simulink model "BAM"  (R2025b)
settings: Solver=FixedStepAuto  StartTime=0.0  StopTime=SimPar.model_params.stop_time  RelTol=1e-3
libraries: simulink x1, ros2lib x1
settings Model: Creator=macheson  LastModifiedBy=Ethan Dueck

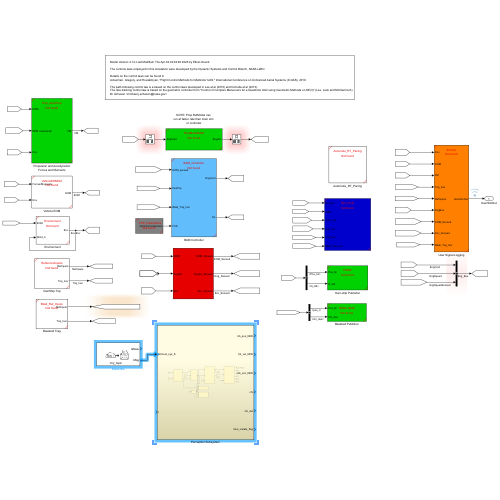
[thumbnail: Simulink's stored preview of the top-level diagram]
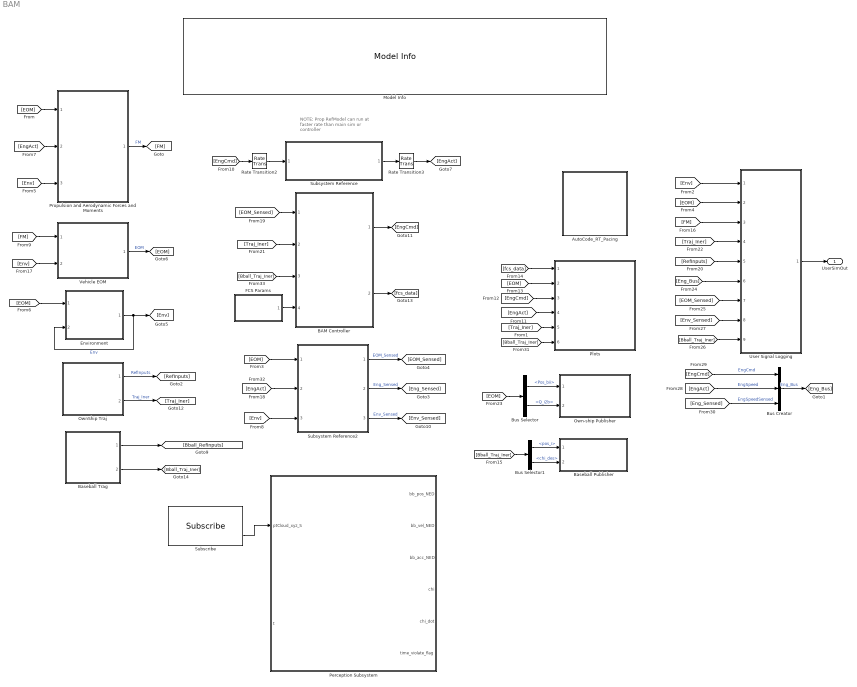
== system BAM ==
  note: NOTE: Prop RefModel can
      | run at faster rate than main sim
      | or controller
  AutoCode_RT_Pacing : Subsystem  ReferencedSubsystem=Autocode_RT_Pacing
  BAM Controller : Subsystem  ReferencedSubsystem=BAM_Controller
  Baseball Publisher : Subsystem  ReferencedSubsystem=ROS2_Bball
  Baseball Trag : Subsystem  ReferencedSubsystem=Bball_Ref_Inputs
  Bus Creator : BusCreator  Inputs=3  OutDataTypeStr=Bus: BUS_PROP_CMD
  Bus Selector : BusSelector  OutputSignals=InertialData.Pos_bii,InertialData.Q_i2b
  Bus Selector1 : BusSelector  OutputSignals=pos_i,chi_des
  Environment : Subsystem  ReferencedSubsystem=Environment
  FCS Params : Subsystem  ReferencedSubsystem=FCS_Parameters
  Model Info : simulink/Model-Wide Utilities/Model Info  Frame=on  DisplayStringWithTags=|  HorizontalTextAlignment=Left  LeftAlignmentValue=0.02
      | Model Version %<ModelVersion>; Last Modified: %<LastModificationDate> by %<LastModifiedBy>
      | 
      | The controls laws employed in this simulation were developed by the Dynamic Systems and Control Branch, NASA LaRC.
      | 
      | Details on the control laws can be found in
      | Ackerman, Gregory, and Hovakimyan, "Flight Control Methods for Multirotor UAS," International Conference on Unmanned Aerial Systems (ICUAS), 2019.
      | 
      | The path-following control law is a based on the control laws developed in Lee et al (2010) and Cichella et al (2013). 
      | The rate-tracking control law is based on the geometric controller from "Control of Complex Maneuvers for a Quadrotor UAV using Geometric Methods on SE(3)" (Lee, Leok and McClamroch)
      | M. Acheson <michael.j.acheson@nasa.gov>
  Own-ship Publisher : Subsystem  ReferencedSubsystem=ROS2
  OwnShip Traj : Subsystem  ReferencedSubsystem=ReferenceInputs
  Perception Subsystem : Subsystem
  Plots : Subsystem  ReferencedSubsystem=Sim_Plots
  Propulsion and Aerodynamic Forces and Moments : Subsystem  ReferencedSubsystem=Poly_AeroProp
  Rate Transition2 : RateTransition  OutPortSampleTime=SimIn.model_params.sim_rate
  Rate Transition3 : RateTransition  OutPortSampleTime=SimIn.model_params.sim_rate
  Subscribe : ros2lib/Subscribe  topicSource=Select from ROS network  topic=/my_topic  messageType=geometry_msgs/Point  sampleTime=-1  QOSHistory=Keep last  QOSDepth=10  QOSReliability=Reliable  QOSDurability=Volatile  QOSDeadline=Inf  QOSLifespan=Inf  QOSLiveliness=Automatic  QOSLeaseDuration=Inf  QOSAvoidROSNamespaceConventions=off
  Subsystem Reference : Subsystem  ReferencedSubsystem=PropModelBAM
  Subsystem Reference2 : Subsystem  ReferencedSubsystem=Sensors
  User Signal Logging : Subsystem  ReferencedSubsystem=SimOut
  Vehicle EOM : Subsystem  ReferencedSubsystem=VehicleEOMRef
  UserSimOut : Outport
  wires:
  Vehicle EOM/1 -> [EOM]  "EOM"
  [FM] -> Vehicle EOM/1
  [Env] -> Vehicle EOM/2
  [EOM] -> Propulsion and Aerodynamic Forces and Moments/1
  OwnShip Traj/1 -> [RefInputs]  "RefInputs"
  Propulsion and Aerodynamic Forces and Moments/1 -> [FM]  "FM"
  [EOM] -> Subsystem Reference2/1
  Environment/1 -> Environment/2, [Env]  "Env"
  [EOM] -> Environment/1
  Subsystem Reference/1 -> Rate Transition3/1
  [EngCmd] -> Rate Transition2/1
  [EngAct] -> Plots/4
  [EngCmd] -> Plots/3
  [EOM] -> Plots/2
  [fcs_data] -> Plots/1
  [EngAct] -> Propulsion and Aerodynamic Forces and Moments/2
  Rate Transition2/1 -> Subsystem Reference/1
  Rate Transition3/1 -> [EngAct]
  Subsystem Reference2/2 -> [Eng_Sensed]  "Eng_Sensed"
  Subsystem Reference2/3 -> [Env_Sensed]  "Env_Sensed"
  [Env] -> Subsystem Reference2/3
  [EngAct] -> Subsystem Reference2/2
  Subsystem Reference2/1 -> [EOM_Sensed]  "EOM_Sensed"
  FCS Params/1 -> BAM Controller/4
  [EOM_Sensed] -> BAM Controller/1
  [Traj_Iner] -> BAM Controller/2
  BAM Controller/1 -> [EngCmd]
  OwnShip Traj/2 -> [Traj_Iner]  "Traj_Iner"
  BAM Controller/2 -> [fcs_data]
  [Env] -> User Signal Logging/1
  [EOM] -> User Signal Logging/2
  [Env_Sensed] -> User Signal Logging/8
  [EOM_Sensed] -> User Signal Logging/7
  [Eng_Bus] -> User Signal Logging/6
  [Traj_Iner] -> User Signal Logging/4
  [RefInputs] -> User Signal Logging/5
  [FM] -> User Signal Logging/3
  Bus Creator/1 -> [Eng_Bus]  "Eng_Bus"
  [Eng_Sensed] -> Bus Creator/3  "EngSpeedSensed"
  [EngAct] -> Bus Creator/2  "EngSpeed"
  [EngCmd] -> Bus Creator/1  "EngCmd"
  [EOM] -> Bus Selector/1
  Bus Selector/1 -> Own-ship Publisher/1  "<Pos_bii>"
  Bus Selector/2 -> Own-ship Publisher/2  "<Q_i2b>"
  User Signal Logging/1 -> UserSimOut/1
  [Traj_Iner] -> Plots/5
  Baseball Trag/1 -> [Bball_RefInputs]
  Baseball Trag/2 -> [Bball_Traj_Iner]
  [Bball_Traj_Iner] -> Plots/6
  [Bball_Traj_Iner] -> User Signal Logging/9
  [Bball_Traj_Iner] -> Bus Selector1/1
  Bus Selector1/1 -> Baseball Publisher/1  "<pos_i>"
  Bus Selector1/2 -> Baseball Publisher/2  "<chi_des>"
  [Env] -> Propulsion and Aerodynamic Forces and Moments/3
  [Bball_Traj_Iner] -> BAM Controller/3
  Subscribe/2 -> Perception Subsystem/1(ptCloud_xyz_S)

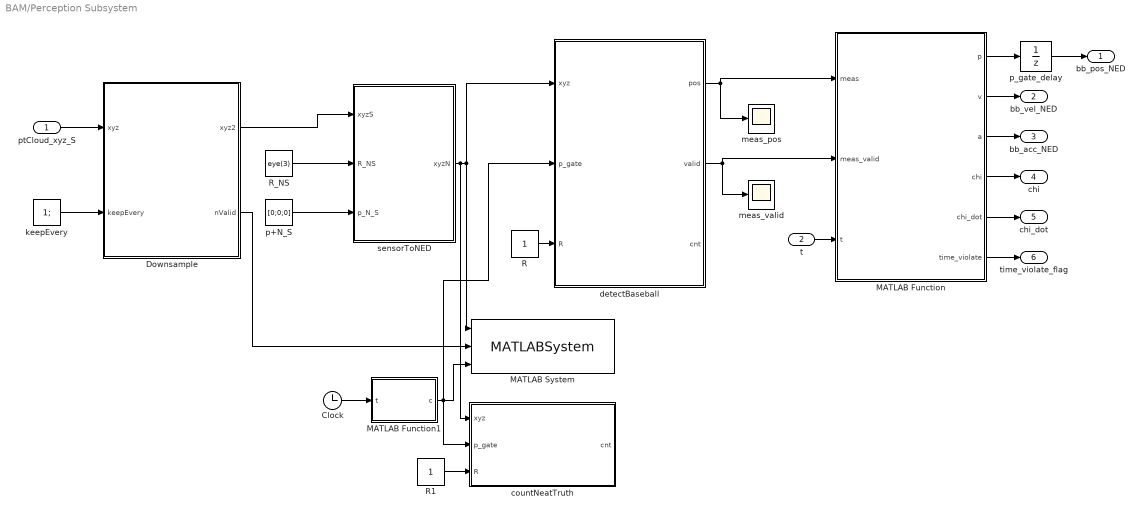
== system BAM/Perception Subsystem ==
  ptCloud_xyz_S : Inport
  t : Inport  Port=2
  Clock : Clock
  Downsample : MATLAB Function  TreatAsAtomicUnit=on
  MATLAB Function : MATLAB Function  TreatAsAtomicUnit=on
  MATLAB Function1 : MATLAB Function  TreatAsAtomicUnit=on
  MATLAB System : MATLABSystem  System=PointCloudViewer  PointSize=3  XLim=[0 60]  YLim=[-30 30]  ZLim=[-10 10]  Decimate=5  ShowDetection=on  SimulateUsing=Interpreted execution
      mask Type: PointCloudViewer
  R : Constant
  R1 : Constant
  R_NS : Constant  Value=eye(3)
  countNeatTruth : MATLAB Function  TreatAsAtomicUnit=on
  detectBaseball : MATLAB Function  TreatAsAtomicUnit=on
  keepEvery : Constant  Value=1;
  meas_pos : Scope
      settings: ActiveDisplayYMinimum=-16.997474195338938  ActiveDisplayYMaximum=39.269494336463588
  meas_valid : Scope
      settings: ActiveDisplayYMinimum=0.9  ActiveDisplayYMaximum=1.1  DataLoggingVariableName=ScopeData4
  p+N_S : Constant  Value=[0;0;0]
  p_gate_delay : UnitDelay  InitialCondition=[10; 0; -2]  SampleTime=-1  HasFrameUpgradeWarning=on
  sensorToNED : MATLAB Function  TreatAsAtomicUnit=on
  bb_pos_NED : Outport
  bb_vel_NED : Outport  Port=2
  bb_acc_NED : Outport  Port=3
  chi : Outport  Port=4
  chi_dot : Outport  Port=5
  time_violate_flag : Outport  Port=6
  wires:
  MATLAB Function/2(v) -> bb_vel_NED/1
  MATLAB Function/3(a) -> bb_acc_NED/1
  MATLAB Function/4(chi) -> chi/1
  MATLAB Function/5(chi_dot) -> chi_dot/1
  MATLAB Function/6(time_violate) -> time_violate_flag/1
  t/1 -> MATLAB Function/3(t)
  detectBaseball/2(valid) -> MATLAB Function/2(meas_valid), meas_valid/1
  R_NS/1 -> sensorToNED/2(R_NS)
  ptCloud_xyz_S/1 -> Downsample/1(xyz)
  Downsample/1(xyz2) -> sensorToNED/1(xyzS)
  keepEvery/1 -> Downsample/2(keepEvery)
  p+N_S/1 -> sensorToNED/3(p_N_S)
  MATLAB Function/1(p) -> p_gate_delay/1
  p_gate_delay/1 -> bb_pos_NED/1
  sensorToNED/1(xyzN) -> countNeatTruth/1(xyz), detectBaseball/1(xyz), MATLAB System/1
  Downsample/2(nValid) -> MATLAB System/2
  detectBaseball/1(pos) -> meas_pos/1, MATLAB Function/1(meas)
  Clock/1 -> MATLAB Function1/1(t)
  MATLAB Function1/1(c) -> detectBaseball/2(p_gate), countNeatTruth/2(p_gate), MATLAB System/3
  R/1 -> detectBaseball/3(R)
  R1/1 -> countNeatTruth/3(R)

== matlab function BAM/Perception Subsystem/sensorToNED ==
  data: xyzS input; xyzN output; R_NS input; p_N_S input
function xyzN = sensorToNED(xyzS, R_NS, p_N_S)
%#codegen
N = size(xyzS,1);
xyzN = zeros(N,3,'like',xyzS);

for i = 1:N
    p = xyzS(i,:).';
    if ~all(isfinite(p))
        xyzN(i,:) = [NaN NaN NaN];
    else
        q = R_NS*p + p_N_S;
        xyzN(i,:) = q.';
    end
end
end

== matlab function BAM/Perception Subsystem/Downsample ==
  data: xyz input; xyz2 output; keepEvery input; nValid output
function [xyz2, nValid] = Downsample(xyz, keepEvery)
%#codegen
N = int32(size(xyz,1));          % should be 11520
xyz2 = zeros(double(N),3,'like',xyz);

nValid = int32(0);

k = int32(keepEvery);
if k < 1
    k = int32(1);
end

% Fill with NaNs (viewer will drop them; avoids axis blow-up)
nanv = cast(NaN,'like',xyz);
xyz2(:,:) = nanv;

j = int32(0);
for i = int32(1):k:N
    j = j + 1;
    xyz2(double(j),:) = xyz(double(i),:);
end

nValid = j;
end

== matlab function BAM/Perception Subsystem/MATLAB Function1 ==
  data: t input; c output
function c = ballTruth(t)
%#codegen
c = [30; 0.5*t; -2];
end

== matlab function BAM/Perception Subsystem/countNeatTruth ==
  data: xyz input; cnt output; p_gate input; R input
function cnt = countNearTruth(xyz, p_gate, R)
%#codegen
cnt = int32(0);
R2 = double(R)*double(R);

N = size(xyz,1);
for i = 1:N
    n = xyz(i,1); e = xyz(i,2); d = xyz(i,3);
    if ~isfinite(n) || ~isfinite(e) || ~isfinite(d)
        continue;
    end
    dn = n - p_gate(1);
    de = e - p_gate(2);
    dd = d - p_gate(3);
    if (dn*dn + de*de + dd*dd) <= R2
        cnt = cnt + 1;
    end
end
end

== matlab function BAM/Perception Subsystem/detectBaseball ==
  data: xyz input; pos output; valid output; cnt output; p_gate input; R input
function [pos, valid, cnt] = detectBallSphereGate(xyz, p_gate, R)
%#codegen
pos   = zeros(3,1);
valid = false;
cnt   = int32(0);

R2 = double(R)*double(R);
s  = zeros(3,1);

N = size(xyz,1);
for i = 1:N
    n = xyz(i,1); e = xyz(i,2); d = xyz(i,3);
    if ~isfinite(n) || ~isfinite(e) || ~isfinite(d)
        continue;
    end

    dn = n - p_gate(1);
    de = e - p_gate(2);
    dd = d - p_gate(3);

    if (dn*dn + de*de + dd*dd) <= R2
        cnt = cnt + 1;
        s = s + [n; e; d];
    end
end

if cnt >= 5
    pos = s / double(cnt);
    valid = true;
end
end

== matlab function BAM/Perception Subsystem/MATLAB Function ==
  data: meas input; p output; meas_valid input; t input; v output; a output; chi output; chi_dot output; time_violate output
function [p,v,a,chi,chi_dot,time_violate] = trackBaseball(meas, meas_valid, t)
%#codegen

persistent p_hat v_hat a_hat t_last t_meas_last init

if isempty(init)
    p_hat = zeros(3,1);
    v_hat = zeros(3,1);
    a_hat = zeros(3,1);
    t_last = t;
    t_meas_last = t;     % <-- avoid -Inf
    init = true;
end

% Guard against time going backwards or being constant
dt_raw = t - t_last;
if ~isfinite(dt_raw) || dt_raw <= 0
    dt = 1e-3;
else
    dt = dt_raw;
end
t_last = t;

% prediction
p_hat = p_hat + v_hat*dt + 0.5*a_hat*(dt*dt);
v_hat = v_hat + a_hat*dt;

% update (alpha-beta-gamma)
alpha = 0.7; beta = 0.2; gamma = 0.05;

meas_ok = meas_valid && all(isfinite(meas(:)));

if meas_ok
    r = meas - p_hat;
    p_hat = p_hat + alpha*r;
    v_hat = v_hat + (beta/dt)*r;
    a_hat = a_hat + (2*gamma/(dt*dt))*r;
    t_meas_last = t;
end

% outputs
p = p_hat; v = v_hat; a = a_hat;

% chi, chi_dot in NED horizontal plane (N=x, E=y)
vn = v(1); ve = v(2);
an = a(1); ae = a(2);

chi = atan2(ve, vn);
chi_dot = (vn*ae - ve*an) / (vn*vn + ve*ve + 1e-6);

% flag if no measurement for too long
age = t - t_meas_last;
if ~isfinite(age) || age < 0
    age = 0;
end
time_violate = age > 0.25;
end
